simulink model "Model_Cosim"  (R2019a)
settings: Solver=VariableStepAuto  StartTime=0.0  StopTime=inf  RelTol=1e-3
values from neighbouring files (symbols this model uses):
  Channel_Delay = 10    [Model_Settings.m]
  Channel_Err_Prob = 0.02    [Model_Settings.m]
  Clock_Freq = 20 * 10^6    (= 20000000)    [Model_Settings.m]
  Data_Rate = Clock_Freq/10    (= 2000000)    [Model_Settings.m]
  Image = zeros(Image_Hight, Image_Width)    [Create_Image.m]    (also in Model_Settings.m = reshape(Image',[1, Hight*Width]))
  Intererence_Error_Probability = 0.5    [Model_Settings.m]
  Intererence_Mean_Period = 1500    [Model_Settings.m]
undefined symbols (not defined in the file or in its folder): gray, Hight, Width
libraries: xbsIndex_r4 x21, commrandsrc3 x4, simulink x2, dspswit3 x2, dspbuff3 x2
settings Model: Creator=User  LastModifiedBy=User

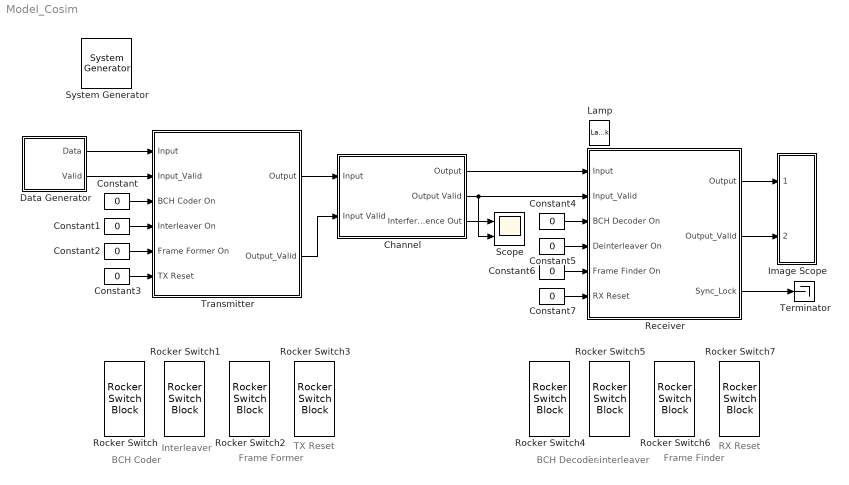
== system Model_Cosim ==
  note: BCH
      | Coder
  note: Interleaver
  note: Frame
      | Former
  note: TX Reset
  note: RX Reset
  note: Deinterleaver
  note: BCH
      | Decoder
  note: Frame
      | Finder
  " System Generator" : xbsIndex_r4/ System Generator  Tag=genX  xilinxfamily=zynquplus  part=xczu9eg  speed=-2-e  package=ffvb1156  synthesis_tool=Vivado  clock_wrapper=Clock Enables  directory=./netlist  proj_type=Vivado  Synth_file=Vivado Synthesis Defaults  Impl_file=Vivado Implementation Defaults  testbench=off  simulink_period=1/Clock_Freq  sysclk_period=1/Clock_Freq*10^9  dcm_input_clock_period=10  incr_netlist=off  trim_vbits=Everywhere in SubSystem  dbl_ovrd=According to Block Masks  core_generation=According to Block Masks  run_coregen=off  deprecated_control=off  eval_field=0  block_type=sysgen
  Channel : Subsystem
  Constant{,1..7} (8 alike) : Constant  Value=0
  Data Generator : Subsystem
  Image Scope : Subsystem
  Lamp : LampBlock  LabelPosition=Hide
  Receiver : Subsystem
  Rocker Switch{,1..7} (8 alike) : RockerSwitchBlock  LabelPosition=Hide
      settings: Values={{'Off', 'On'}, [0 1]}
  Scope : Scope  NumInputPorts=2
  Terminator : Terminator
  Transmitter : Subsystem
  wires:
  Receiver/3(Sync_Lock) -> Terminator/1
  Data Generator/1(Data) -> Transmitter/1(Input)
  Data Generator/2(Valid) -> Transmitter/2(Input_Valid)
  Receiver/1(Output) -> Image Scope/1(Data)
  Receiver/2(Output_Valid) -> Image Scope/2(Valid)
  Transmitter/1(Output) -> Channel/1(Input)
  Transmitter/2(Output_Valid) -> Channel/2(Input Valid)
  Channel/1(Output) -> Receiver/1(Input)
  Channel/2(Output Valid) -> Scope/2, Receiver/2(Input_Valid)
  Constant/1 -> Transmitter/3(BCH Coder On)
  Constant1/1 -> Transmitter/4(Interleaver On)
  Constant2/1 -> Transmitter/5(Frame Former On)
  Constant3/1 -> Transmitter/6(TX Reset)
  Constant4/1 -> Receiver/3(BCH Decoder On)
  Constant5/1 -> Receiver/4(Deinterleaver On)
  Constant6/1 -> Receiver/5(Frame Finder On)
  Constant7/1 -> Receiver/6(RX Reset)
  Channel/3(Interference Out) -> Scope/1

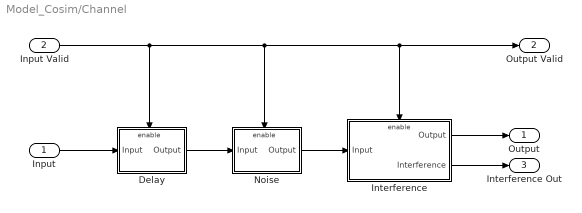
== system Model_Cosim/Channel ==
  Input : Inport
  Input Valid : Inport  Port=2
  Delay : Subsystem
  Interference : Subsystem
  Noise : Subsystem
  Output : Outport
  Output Valid : Outport  Port=2
  Interference Out : Outport  Port=3
  wires:
  Input Valid/1 -> Noise/Enable, Interference/Enable, Output Valid/1, Delay/Enable
  Input/1 -> Delay/1(Input)
  Delay/1(Output) -> Noise/1(Input)
  Noise/1(Output) -> Interference/1(Input)
  Interference/1(Output) -> Output/1
  Interference/2(Interference) -> Interference Out/1

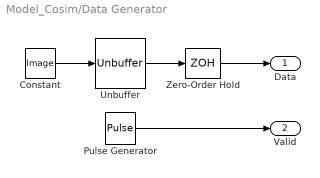
== system Model_Cosim/Data Generator ==
  Constant : Constant  Value=Image  SampleTime=Hight*Width/Data_Rate
  Pulse Generator : DiscretePulseGenerator  Period=Clock_Freq/Data_Rate  SampleTime=1/Clock_Freq
  Unbuffer : Unbuffer
  Zero-Order Hold : ZeroOrderHold  SampleTime=1/Clock_Freq
  Data : Outport
  Valid : Outport  Port=2
  wires:
  Constant/1 -> Unbuffer/1
  Unbuffer/1 -> Zero-Order Hold/1
  Zero-Order Hold/1 -> Data/1
  Pulse Generator/1 -> Valid/1

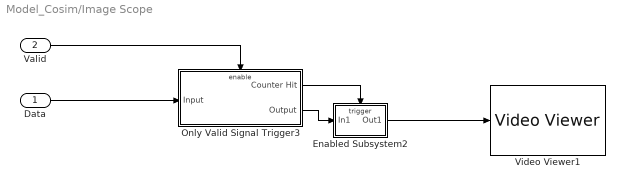
== system Model_Cosim/Image Scope ==
  Data : Inport
  Valid : Inport  Port=2
  Enabled Subsystem2 : Subsystem  TreatAsAtomicUnit=on
  Only Valid Signal Trigger3 : Subsystem  TreatAsAtomicUnit=on
  Video Viewer1 : VideoViewer  colormapValue=gray(256)  FigPos=[1102 971 609 713]
  wires:
  Enabled Subsystem2/1(Out1) -> Video Viewer1/1
  Only Valid Signal Trigger3/2(Output) -> Enabled Subsystem2/1(In1)
  Valid/1 -> Only Valid Signal Trigger3/Enable
  Only Valid Signal Trigger3/1(Counter Hit) -> Enabled Subsystem2/Trigger
  Data/1 -> Only Valid Signal Trigger3/1(Input)

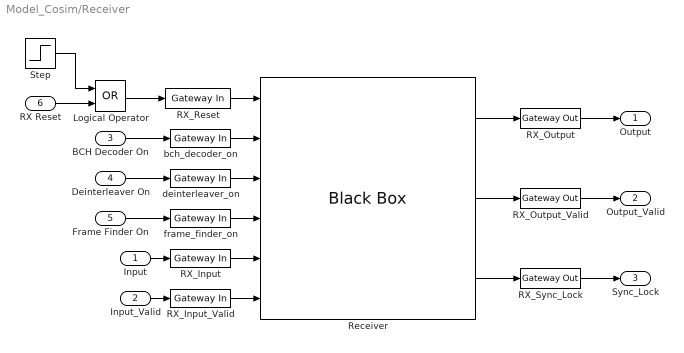
== system Model_Cosim/Receiver ==
  Input : Inport
  Input_Valid : Inport  Port=2
  BCH Decoder On : Inport  Port=3
  Deinterleaver On : Inport  Port=4
  Frame Finder On : Inport  Port=5
  RX Reset : Inport  Port=6
  Logical Operator : Logic  Operator=OR  AllPortsSameDT=off  OutDataTypeStr=boolean
  RX_Input : xbsIndex_r4/Gateway In  gui_display_data_type=Fixed-point  arith_type=Unsigned  n_bits=1  bin_pt=0  preci_type=Single  exp_width=8  frac_width=24  rows=1  columns=1  quantization="Round  (unbiased: +/- Inf)"  overflow=Saturate  period=1/Clock_Freq  UseAsADC=off  ADCChannel='1'  interface=None  automatic_assignment=on  address_offset=hex2dec('00')  intf_name=''  intf_description=''  default_value=0  timing_constraint=None  locs_specified=off  LOCs={}  io_standard={}  inherit_from_input=off  hdl_port=on  dbl_ovrd=off  block_type=gatewayin
  RX_Input_Valid : xbsIndex_r4/Gateway In  gui_display_data_type=Fixed-point  arith_type=Unsigned  n_bits=1  bin_pt=0  preci_type=Single  exp_width=8  frac_width=24  rows=1  columns=1  quantization="Round  (unbiased: +/- Inf)"  overflow=Saturate  period=1/Clock_Freq  UseAsADC=off  ADCChannel='1'  interface=None  automatic_assignment=on  address_offset=hex2dec('00')  intf_name=''  intf_description=''  default_value=0  timing_constraint=None  locs_specified=off  LOCs={}  io_standard={}  inherit_from_input=off  hdl_port=on  dbl_ovrd=off  block_type=gatewayin
  RX_Output : xbsIndex_r4/Gateway Out  inherit_from_input=off  hdl_port=on  rows=1  columns=1  UseAsDAC=off  DACChannel='1'  interface=None  automatic_assignment=on  address_offset=hex2dec('00')  intf_name=''  intf_description=''  timing_constraint=None  locs_specified=off  LOCs={}  io_standard={}  block_type=gatewayout
  RX_Output_Valid : xbsIndex_r4/Gateway Out  inherit_from_input=off  hdl_port=on  rows=1  columns=1  UseAsDAC=off  DACChannel='1'  interface=None  automatic_assignment=on  address_offset=hex2dec('00')  intf_name=''  intf_description=''  timing_constraint=None  locs_specified=off  LOCs={}  io_standard={}  block_type=gatewayout
  RX_Reset : xbsIndex_r4/Gateway In  gui_display_data_type=Boolean  arith_type=Boolean  n_bits=16  bin_pt=14  preci_type=Single  exp_width=8  frac_width=24  rows=1  columns=1  quantization="Round  (unbiased: +/- Inf)"  overflow=Saturate  period=1/Clock_Freq  UseAsADC=off  ADCChannel='1'  interface=None  automatic_assignment=on  address_offset=hex2dec('00')  intf_name=''  intf_description=''  default_value=0  timing_constraint=None  locs_specified=off  LOCs={}  io_standard={}  inherit_from_input=off  hdl_port=on  dbl_ovrd=off  block_type=gatewayin
  RX_Sync_Lock : xbsIndex_r4/Gateway Out  inherit_from_input=off  hdl_port=on  rows=1  columns=1  UseAsDAC=off  DACChannel='1'  interface=None  automatic_assignment=on  address_offset=hex2dec('00')  intf_name=''  intf_description=''  timing_constraint=None  locs_specified=off  LOCs={}  io_standard={}  block_type=gatewayout
  Receiver : xbsIndex_r4/Black Box  init_code=Receiver_config  sim_method=ISE Simulator  verbose=off  block_type=blackbox2
  Step : Step  Time=300/Clock_Freq  Before=1  After=0  SampleTime=1/Clock_Freq
  bch_decoder_on : xbsIndex_r4/Gateway In  gui_display_data_type=Fixed-point  arith_type=Unsigned  n_bits=1  bin_pt=0  preci_type=Single  exp_width=8  frac_width=24  rows=1  columns=1  quantization="Round  (unbiased: +/- Inf)"  overflow=Saturate  period=1/Clock_Freq  UseAsADC=off  ADCChannel='1'  interface=None  automatic_assignment=on  address_offset=hex2dec('00')  intf_name=''  intf_description=''  default_value=0  timing_constraint=None  locs_specified=off  LOCs={}  io_standard={}  inherit_from_input=off  hdl_port=on  dbl_ovrd=off  block_type=gatewayin
  deinterleaver_on : xbsIndex_r4/Gateway In  gui_display_data_type=Fixed-point  arith_type=Unsigned  n_bits=1  bin_pt=0  preci_type=Single  exp_width=8  frac_width=24  rows=1  columns=1  quantization="Round  (unbiased: +/- Inf)"  overflow=Saturate  period=1/Clock_Freq  UseAsADC=off  ADCChannel='1'  interface=None  automatic_assignment=on  address_offset=hex2dec('00')  intf_name=''  intf_description=''  default_value=0  timing_constraint=None  locs_specified=off  LOCs={}  io_standard={}  inherit_from_input=off  hdl_port=on  dbl_ovrd=off  block_type=gatewayin
  frame_finder_on : xbsIndex_r4/Gateway In  gui_display_data_type=Fixed-point  arith_type=Unsigned  n_bits=1  bin_pt=0  preci_type=Single  exp_width=8  frac_width=24  rows=1  columns=1  quantization="Round  (unbiased: +/- Inf)"  overflow=Saturate  period=1/Clock_Freq  UseAsADC=off  ADCChannel='1'  interface=None  automatic_assignment=on  address_offset=hex2dec('00')  intf_name=''  intf_description=''  default_value=0  timing_constraint=None  locs_specified=off  LOCs={}  io_standard={}  inherit_from_input=off  hdl_port=on  dbl_ovrd=off  block_type=gatewayin
  Output : Outport
  Output_Valid : Outport  Port=2
  Sync_Lock : Outport  Port=3
  wires:
  RX_Sync_Lock/1 -> Sync_Lock/1
  Receiver/2 -> RX_Output_Valid/1
  RX_Output/1 -> Output/1
  RX_Input/1 -> Receiver/5
  RX_Input_Valid/1 -> Receiver/6
  Input_Valid/1 -> RX_Input_Valid/1
  Receiver/3 -> RX_Sync_Lock/1
  Receiver/1 -> RX_Output/1
  RX_Reset/1 -> Receiver/1
  Input/1 -> RX_Input/1
  RX_Output_Valid/1 -> Output_Valid/1
  Deinterleaver On/1 -> deinterleaver_on/1
  deinterleaver_on/1 -> Receiver/3
  frame_finder_on/1 -> Receiver/4
  bch_decoder_on/1 -> Receiver/2
  BCH Decoder On/1 -> bch_decoder_on/1
  Frame Finder On/1 -> frame_finder_on/1
  Logical Operator/1 -> RX_Reset/1
  RX Reset/1 -> Logical Operator/2
  Step/1 -> Logical Operator/1

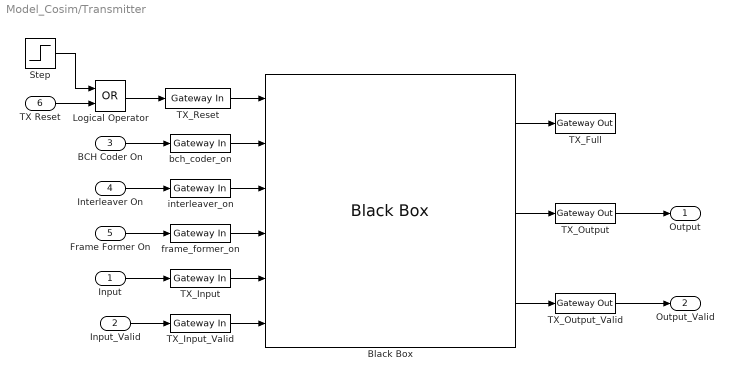
== system Model_Cosim/Transmitter ==
  Input : Inport
  Input_Valid : Inport  Port=2
  BCH Coder On : Inport  Port=3
  Interleaver On : Inport  Port=4
  Frame Former On : Inport  Port=5
  TX Reset : Inport  Port=6
  Black Box : xbsIndex_r4/Black Box  init_code=Transmitter_config  sim_method=ISE Simulator  verbose=off  block_type=blackbox2
  Logical Operator : Logic  Operator=OR  AllPortsSameDT=off  OutDataTypeStr=boolean
  Step : Step  Time=300/Clock_Freq  Before=1  After=0  SampleTime=1/Clock_Freq
  TX_Full : xbsIndex_r4/Gateway Out  inherit_from_input=off  hdl_port=on  rows=1  columns=1  UseAsDAC=off  DACChannel='1'  interface=None  automatic_assignment=on  address_offset=hex2dec('00')  intf_name=''  intf_description=''  timing_constraint=None  locs_specified=off  LOCs={}  io_standard={}  block_type=gatewayout
  TX_Input : xbsIndex_r4/Gateway In  gui_display_data_type=Fixed-point  arith_type=Unsigned  n_bits=1  bin_pt=0  preci_type=Single  exp_width=8  frac_width=24  rows=1  columns=1  quantization="Round  (unbiased: +/- Inf)"  overflow=Saturate  period=1/Clock_Freq  UseAsADC=off  ADCChannel='1'  interface=None  automatic_assignment=on  address_offset=hex2dec('00')  intf_name=''  intf_description=''  default_value=0  timing_constraint=None  locs_specified=off  LOCs={}  io_standard={}  inherit_from_input=off  hdl_port=on  dbl_ovrd=off  block_type=gatewayin
  TX_Input_Valid : xbsIndex_r4/Gateway In  gui_display_data_type=Fixed-point  arith_type=Unsigned  n_bits=1  bin_pt=0  preci_type=Single  exp_width=8  frac_width=24  rows=1  columns=1  quantization="Round  (unbiased: +/- Inf)"  overflow=Saturate  period=1/Clock_Freq  UseAsADC=off  ADCChannel='1'  interface=None  automatic_assignment=on  address_offset=hex2dec('00')  intf_name=''  intf_description=''  default_value=0  timing_constraint=None  locs_specified=off  LOCs={}  io_standard={}  inherit_from_input=off  hdl_port=on  dbl_ovrd=off  block_type=gatewayin
  TX_Output : xbsIndex_r4/Gateway Out  inherit_from_input=off  hdl_port=on  rows=1  columns=1  UseAsDAC=off  DACChannel='1'  interface=None  automatic_assignment=on  address_offset=hex2dec('00')  intf_name=''  intf_description=''  timing_constraint=None  locs_specified=off  LOCs={}  io_standard={}  block_type=gatewayout
  TX_Output_Valid : xbsIndex_r4/Gateway Out  inherit_from_input=off  hdl_port=on  rows=1  columns=1  UseAsDAC=off  DACChannel='1'  interface=None  automatic_assignment=on  address_offset=hex2dec('00')  intf_name=''  intf_description=''  timing_constraint=None  locs_specified=off  LOCs={}  io_standard={}  block_type=gatewayout
  TX_Reset : xbsIndex_r4/Gateway In  gui_display_data_type=Boolean  arith_type=Boolean  n_bits=16  bin_pt=14  preci_type=Single  exp_width=8  frac_width=24  rows=1  columns=1  quantization="Round  (unbiased: +/- Inf)"  overflow=Saturate  period=1/Clock_Freq  UseAsADC=off  ADCChannel='1'  interface=None  automatic_assignment=on  address_offset=hex2dec('00')  intf_name=''  intf_description=''  default_value=0  timing_constraint=None  locs_specified=off  LOCs={}  io_standard={}  inherit_from_input=off  hdl_port=on  dbl_ovrd=off  block_type=gatewayin
  bch_coder_on : xbsIndex_r4/Gateway In  gui_display_data_type=Fixed-point  arith_type=Unsigned  n_bits=1  bin_pt=0  preci_type=Single  exp_width=8  frac_width=24  rows=1  columns=1  quantization="Round  (unbiased: +/- Inf)"  overflow=Saturate  period=1/Clock_Freq  UseAsADC=off  ADCChannel='1'  interface=None  automatic_assignment=on  address_offset=hex2dec('00')  intf_name=''  intf_description=''  default_value=0  timing_constraint=None  locs_specified=off  LOCs={}  io_standard={}  inherit_from_input=off  hdl_port=on  dbl_ovrd=off  block_type=gatewayin
  frame_former_on : xbsIndex_r4/Gateway In  gui_display_data_type=Fixed-point  arith_type=Unsigned  n_bits=1  bin_pt=0  preci_type=Single  exp_width=8  frac_width=24  rows=1  columns=1  quantization="Round  (unbiased: +/- Inf)"  overflow=Saturate  period=1/Clock_Freq  UseAsADC=off  ADCChannel='1'  interface=None  automatic_assignment=on  address_offset=hex2dec('00')  intf_name=''  intf_description=''  default_value=0  timing_constraint=None  locs_specified=off  LOCs={}  io_standard={}  inherit_from_input=off  hdl_port=on  dbl_ovrd=off  block_type=gatewayin
  interleaver_on : xbsIndex_r4/Gateway In  gui_display_data_type=Fixed-point  arith_type=Unsigned  n_bits=1  bin_pt=0  preci_type=Single  exp_width=8  frac_width=24  rows=1  columns=1  quantization="Round  (unbiased: +/- Inf)"  overflow=Saturate  period=1/Clock_Freq  UseAsADC=off  ADCChannel='1'  interface=None  automatic_assignment=on  address_offset=hex2dec('00')  intf_name=''  intf_description=''  default_value=0  timing_constraint=None  locs_specified=off  LOCs={}  io_standard={}  inherit_from_input=off  hdl_port=on  dbl_ovrd=off  block_type=gatewayin
  Output : Outport
  Output_Valid : Outport  Port=2
  wires:
  TX_Output_Valid/1 -> Output_Valid/1
  Input_Valid/1 -> TX_Input_Valid/1
  TX_Input_Valid/1 -> Black Box/6
  TX_Reset/1 -> Black Box/1
  Black Box/1 -> TX_Full/1
  Black Box/2 -> TX_Output/1
  Input/1 -> TX_Input/1
  TX_Output/1 -> Output/1
  TX_Input/1 -> Black Box/5
  Black Box/3 -> TX_Output_Valid/1
  bch_coder_on/1 -> Black Box/2
  interleaver_on/1 -> Black Box/3
  frame_former_on/1 -> Black Box/4
  BCH Coder On/1 -> bch_coder_on/1
  Interleaver On/1 -> interleaver_on/1
  Frame Former On/1 -> frame_former_on/1
  Step/1 -> Logical Operator/1
  TX Reset/1 -> Logical Operator/2
  Logical Operator/1 -> TX_Reset/1

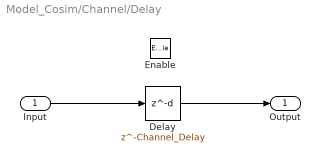
== system Model_Cosim/Channel/Delay ==
  Input : Inport
  Enable : EnablePort
  Delay : Delay  DelayLength=Channel_Delay
  Output : Outport
  wires:
  Input/1 -> Delay/1
  Delay/1 -> Output/1

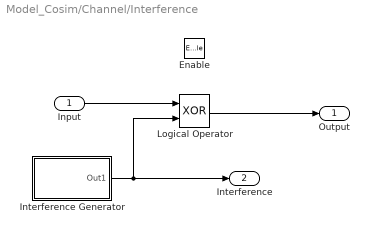
== system Model_Cosim/Channel/Interference ==
  Input : Inport
  Enable : EnablePort
  Interference Generator : Subsystem
  Logical Operator : Logic  Operator=XOR  AllPortsSameDT=off  OutDataTypeStr=boolean
  Output : Outport
  Interference : Outport  Port=2
  wires:
  Input/1 -> Logical Operator/1
  Logical Operator/1 -> Output/1
  Interference Generator/1(Out1) -> Interference/1, Logical Operator/2

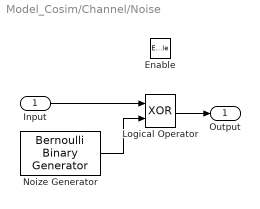
== system Model_Cosim/Channel/Noise ==
  Input : Inport
  Enable : EnablePort
  Logical Operator : Logic  Operator=XOR  AllPortsSameDT=off  OutDataTypeStr=boolean
  Noize Generator : commrandsrc3/Bernoulli Binary Generator  ProbabilityOfZero=1 - Channel_Err_Prob  SeedSource=Auto  Seed=0  SampleTime=1/Clock_Freq  SamplesPerFrame=1  OutputDataType=double  SimulateUsing=Interpreted execution
      settings: SourceProductName=Communications Toolbox
  Output : Outport
  wires:
  Input/1 -> Logical Operator/1
  Logical Operator/1 -> Output/1
  Noize Generator/1 -> Logical Operator/2

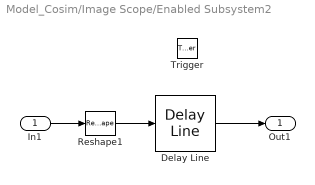
== system Model_Cosim/Image Scope/Enabled Subsystem2 ==
  In1 : Inport
  Trigger : TriggerPort  VariantControl=Variant  PortDimensions=1
  Delay Line : dspbuff3/Delay Line  siz=Hight  ic=0  directfeed=off  enable_output=off  hold_output=off  OutputFrames=off
      settings: SourceProductName=DSP System Toolbox  SourceProductBaseCode=DS
  Reshape1 : Reshape  OutputDimensionality=Row vector (2-D)
  Out1 : Outport
  wires:
  Delay Line/1 -> Out1/1
  Reshape1/1 -> Delay Line/1
  In1/1 -> Reshape1/1

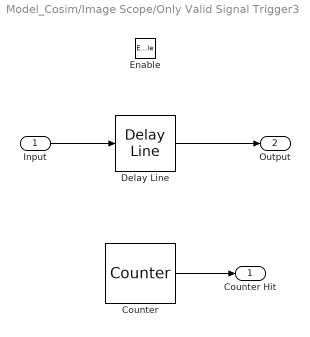
== system Model_Cosim/Image Scope/Only Valid Signal Trigger3 ==
  Input : Inport
  Enable : EnablePort
  Counter : dspswit3/Counter  Direction=Up  CountEvent=Free running  CounterSize=User defined  MaxCount=Width - 1  InitialCount=0  Output=Hit  HitValue=Width - 1  ResetInput=off  SamplesPerFrame=1  Ts=1/Clock_Freq  CntDtype=double  HitDtype=Logical
  Delay Line : dspbuff3/Delay Line  siz=Width  ic=0  directfeed=on  enable_output=off  hold_output=off  OutputFrames=off
      settings: SourceProductName=DSP System Toolbox  SourceProductBaseCode=DS
  Counter Hit : Outport
  Output : Outport  Port=2
  wires:
  Counter/1 -> Counter Hit/1
  Delay Line/1 -> Output/1
  Input/1 -> Delay Line/1

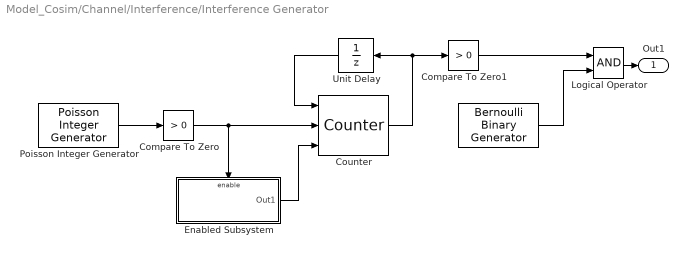
== system Model_Cosim/Channel/Interference/Interference Generator ==
  " " : commrandsrc3/Bernoulli Binary Generator  ProbabilityOfZero=1-Intererence_Error_Probability  SeedSource=Auto  Seed=0  SampleTime=1/Clock_Freq  SamplesPerFrame=1  OutputDataType=double  SimulateUsing=Interpreted execution
      settings: SourceProductName=Communications Toolbox
  Compare To Zero : simulink/Logic and Bit Operations/Compare To Zero  relop=>  OutDataTypeStr=boolean
  Compare To Zero1 : simulink/Logic and Bit Operations/Compare To Zero  relop=>  OutDataTypeStr=boolean
  Counter : dspswit3/Counter  Direction=Up  CountEvent=Non-zero sample  CounterSize=Specify via input port  MaxCount=255  InitialCount=1  Output=Count  HitValue=32  ResetInput=on  SamplesPerFrame=1  Ts=1  CntDtype=uint32  HitDtype=Logical
  Enabled Subsystem : Subsystem  TreatAsAtomicUnit=on
  Logical Operator : Logic  AllPortsSameDT=off  OutDataTypeStr=boolean
  Poisson Integer Generator : commrandsrc3/Poisson Integer Generator  PoissonParameter=1/Intererence_Mean_Period  SeedSource=Auto  Seed=0  SampleTime=1/Clock_Freq  SamplesPerFrame=1  OutputDataType=double  SimulateUsing=Interpreted execution
      settings: SourceProductName=Communications Toolbox  SourceProductBaseCode=CM
  Unit Delay : UnitDelay  SampleTime=-1  HasFrameUpgradeWarning=on
  Out1 : Outport
  wires:
  Poisson Integer Generator/1 -> Compare To Zero/1
  Compare To Zero/1 -> Enabled Subsystem/Enable, Counter/2
  Enabled Subsystem/1(Out1) -> Counter/3
  Unit Delay/1 -> Counter/1
  Counter/1 -> Compare To Zero1/1, Unit Delay/1
  " "/1 -> Logical Operator/2
  Logical Operator/1 -> Out1/1
  Compare To Zero1/1 -> Logical Operator/1

== system Model_Cosim/Channel/Interference/Interference Generator/Enabled Subsystem ==
  Enable : EnablePort
  Random Integer Generator : commrandsrc3/Random Integer Generator  SetSize=Intererence_Max_Width  SeedSource=Auto  Seed=0  SampleTime=1/Clock_Freq  SamplesPerFrame=1  OutputDataType=uint32  SimulateUsing=Interpreted execution
      settings: SourceProductName=Communications Toolbox
  Out1 : Outport
  wires:
  Random Integer Generator/1 -> Out1/1
